simulink model "SCCS_AntiPinch_SM_03"  (R2024a)
settings: Solver=ode3  StartTime=0.0  StopTime=10.0  FixedStep=0.01  RelTol=1e-3
settings Model: Creator=Kishore  LastModifiedBy=Kishore

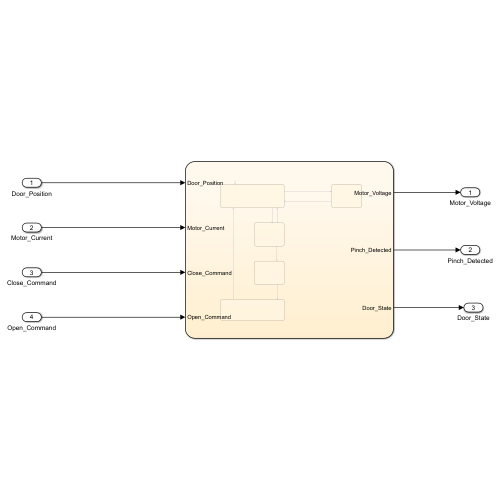
[thumbnail: Simulink's stored preview of the top-level diagram]
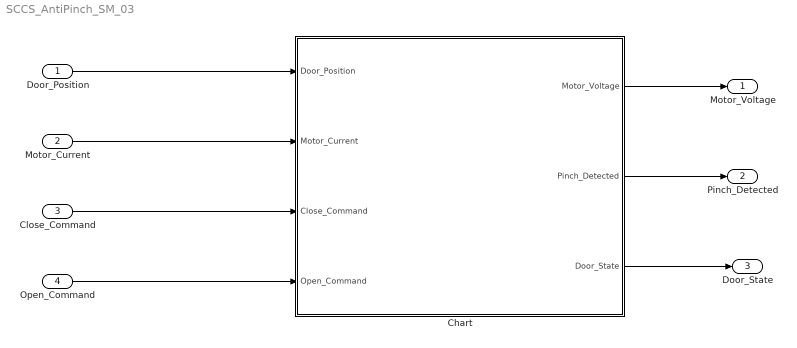
== system SCCS_AntiPinch_SM_03 ==
  Door_Position : Inport
  Motor_Current : Inport  Port=2
  Close_Command : Inport  Port=3
  Open_Command : Inport  Port=4
  Chart : Stateflow chart  TreatAsAtomicUnit=on
  Motor_Voltage : Outport
  Pinch_Detected : Outport  Port=2
  Door_State : Outport  Port=3
  wires:
  Chart/1(Motor_Voltage) -> Motor_Voltage/1
  Chart/2(Pinch_Detected) -> Pinch_Detected/1
  Chart/3(Door_State) -> Door_State/1
  Door_Position/1 -> Chart/1(Door_Position)
  Motor_Current/1 -> Chart/2(Motor_Current)
  Close_Command/1 -> Chart/3(Close_Command)
  Open_Command/1 -> Chart/4(Open_Command)

== stateflow chart SCCS_AntiPinch_SM_03/Chart ==
  state IDLE
    entry :
    Motor_Voltage = 0;
    Pinch_Detected = 0;
    Door_State = 1;
  state OPENING
    entry :
    Motor_Voltage = 10;
    Door_State = 2;
  state CLOSING
    entry :
    Motor_Voltage = -10;
    Door_State = 3;
  state PINCH_DETECTED
    entry :
    Motor_Voltage = 0;
    Pinch_Detected = 1;
    Door_State = 4;
  state REVERSING
    entry :
    Motor_Voltage = 10;
    Door_State = 5;
  (default) -> IDLE
  IDLE -> OPENING [order 1] : [Open_Command == 1]
  OPENING -> IDLE : [Door_Position >= 400 || Open_Command == 0]
  REVERSING -> IDLE : [after(0.5, sec)]
  IDLE -> CLOSING [order 2] : [Close_Command == 1]
  CLOSING -> IDLE [order 2] : [Door_Position <= 0 || Close_Command == 0]
  CLOSING -> PINCH_DETECTED [order 1] : [Motor_Current > 8]
  PINCH_DETECTED -> REVERSING : [after(0.1, sec)]
  data: Door_Position input; Motor_Current input; Close_Command input; Open_Command input; Motor_Voltage output; Pinch_Detected output; Door_State output
